simulink model "test_com_TireLoadEstimator"  (R2017a)
settings: Solver=FixedStepDiscrete  StartTime=450  StopTime=650  FixedStep=0.001  RelTol=1e-3
undefined symbols (not defined in the file or in its folder): GearRatio
settings Model: DataDictionary=controller_dict.sldd  SnapshotInterval=100  Creator=daniel  LastModifiedBy=rieth
settings DataIOCC: ExternalInput=VD_SteeringAngle_Value, VD_V2O_SpeedLongitudinal, VD_V2O_SpeedLateral, PT_Motor_MotorSpeed_FL, PT_Motor_MotorSpeed_FR, PT_Motor_MotorSpeed_RL, PT_Motor_MotorSpeed_RR, VD_Gyro_Front_Accel_X, VD_Gyro_Front_Accel_Y, VD_Gyro_Front_Accel_Z, VD_Gyro_Front_ARate_X, VD_Gyro_Front_ARate_Y, VD_Gyro_Front_ARate_Z, VD_Gyro_Front_Comp_X, VD_Gyro_Front_Comp_Y, VD_Gyro_Front_Comp_Z, VD_Gyro_Front_Temp, VD_Gyro_Rear_Accel_X, VD_Gyro_Rear_Accel_Y, VD_Gyro_Rear_Accel_Z, VD_Gyro_Rear_ARate_X, VD_Gyro_Rear_ARate_Y,VD_Gyro_Rear_ARate_Z, VD_Gyro_Rear_Comp_X, VD_Gyro_Rear_Comp_Y, VD_Gyro_Rear_Comp_Z, VD_Gyro_Rear_Temp,VD_Suspension_Hall_FL,VD_Suspension_Hall_FR,VD_Suspension_Hall_RL,VD_Suspension_Hall_RR  LimitDataPoints=on  LoadExternalInput=on  SaveFormat=Array  SaveOutput=off  SignalLogging=off  DSMLogging=off  SaveTime=off
settings OptimizationCC: DefaultParameterBehavior=Inlined  UseDivisionForNetSlopeComputation=on  StateBitsets=on  DataBitsets=on  LifeSpan=1
settings DebuggingCC: SolverPrmCheckMsg=warning  ParameterPrecisionLossMsg=none  AllowSymbolicDim=off  SFUnexpectedBacktrackingDiag=warning  SFNoUnconditionalDefaultTransitionDiag=warning  SFExecutionAtInitializationDiag=none
settings HardwareCC: ProdBitPerPointer=32  ProdBitPerSizeT=32  ProdBitPerPtrDiffT=32  ProdLargestAtomicInteger=Long  ProdLargestAtomicFloat=Double  ProdWordSize=32  ProdHWDeviceType=Texas Instruments->TMS570 Cortex-R4
settings ModelReferenceCC: PropagateSignalLabelsOutOfModel=off
settings SFSimCC: SimBuildMode=sf_nonincremental_build  MATLABDynamicMemAlloc=off
settings RTWCC: SystemTargetFile=ert.tlc  GenCodeOnly=on  TemplateMakefile=ert_default_tmf  Description=Embedded Coder  GenerateReport=on  BuildConfiguration=Faster Runs  IncludeHyperlinkInReport=on  LaunchReport=on  GenerateTraceReport=on
settings CodeAppCC: IgnoreCustomStorageClasses=off  SFDataObjDesc=on
settings ERTTargetCC: MultiwordLength=2048  GenerateSampleERTMain=on  InlinedParameterPlacement=NonHierarchical  ERTCustomFileTemplate=example_file_process.tlc  ConvertIfToSwitch=off  SuppressUnreachableDefaultCases=off
settings ConfigComp: CovMetricSettings=dw  CovHtmlReporting=on  CovSaveCumulativeToWorkspaceVar=on  CovSaveSingleToWorkspaceVar=on  CovExternalEMLEnable=off  CovSFcnEnable=off
settings ConfigurationSet: Description=SimMechanics 2G

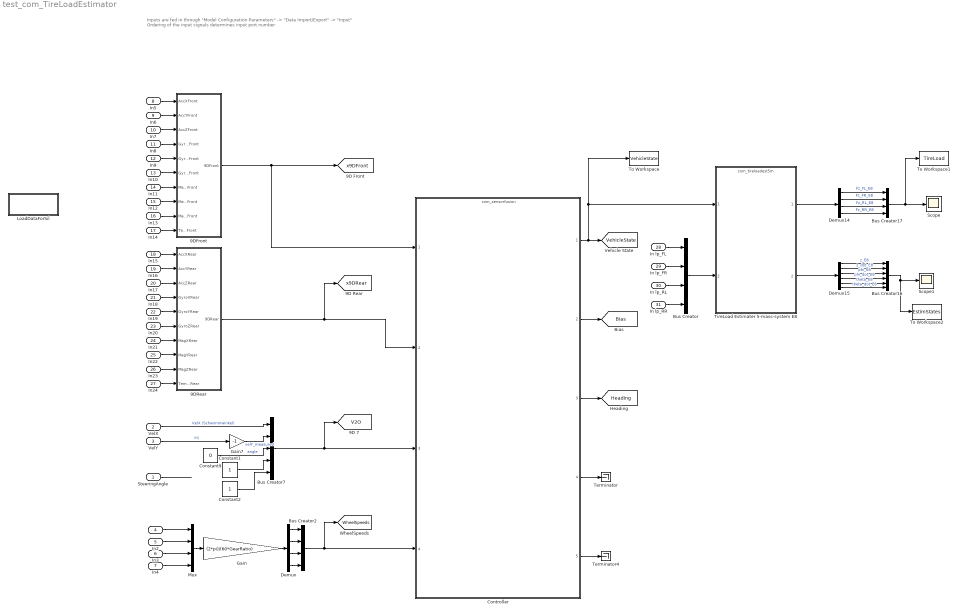
== system test_com_TireLoadEstimator ==
  note: Inputs are fed in through "Model Configuration Parameters" -> "Data Import/Export" -> "Input"
      | Ordering of the input signals determines input port number
  SteeringAngle : Inport  OutDataTypeStr=single  Interpolate=off
  VelX : Inport  Port=2  OutDataTypeStr=single
  VelY : Inport  Port=3  OutDataTypeStr=single
  " " : Inport  Port=4  OutDataTypeStr=single
  In2 : Inport  Port=5  OutDataTypeStr=single
  In3 : Inport  Port=6  OutDataTypeStr=single
  In4 : Inport  Port=7  OutDataTypeStr=single
  In5 : Inport  Port=8
  In6 : Inport  Port=9
  In7 : Inport  Port=10
  In8 : Inport  Port=11
  In9 : Inport  Port=12
  In10 : Inport  Port=13
  In11 : Inport  Port=14
  In12 : Inport  Port=15
  In13 : Inport  Port=16
  In14 : Inport  Port=17
  In15 : Inport  Port=18
  In16 : Inport  Port=19
  In17 : Inport  Port=20
  In18 : Inport  Port=21
  In19 : Inport  Port=22
  In20 : Inport  Port=23
  In21 : Inport  Port=24
  In22 : Inport  Port=25
  In23 : Inport  Port=26
  In24 : Inport  Port=27
  In lp_FL : Inport  Port=28  OutDataTypeStr=single
  In lp_FR : Inport  Port=29  OutDataTypeStr=single
  In lp_RL : Inport  Port=30  OutDataTypeStr=single
  In lp_RR : Inport  Port=31  OutDataTypeStr=single
  9DFront : Subsystem
  9DRear : Subsystem
  Bus Creator : BusCreator  Inputs=4
  Bus Creator16 : BusCreator  Inputs=6
  Bus Creator17 : BusCreator  Inputs=4
  Bus Creator2 : BusCreator  Inputs=4  OutDataTypeStr=Bus: control_WheelSpeed
      settings: InheritFromInputs=off
  Bus Creator7 : BusCreator  Inputs=5  OutDataTypeStr=Bus: control_velocity
      settings: InheritFromInputs=off
  Constant1 : Constant  OutDataTypeStr=boolean
  Constant2 : Constant  OutDataTypeStr=boolean
  Constant9 : Constant  Value=0  OutDataTypeStr=Inherit: Inherit via back propagation
  Controller : ModelReference  ModelNameDialog=com_sensorfusion.slx  SimulationMode=Normal  ModelReferenceVersion=1.1509
  Demux : Demux
  Demux14 : Demux
  Demux15 : Demux  Outputs=6
  Gain : Gain  Gain=(2*pi)/(60*GearRatio)
  Gain7 : Gain  Gain=-1
  LoadDataForSil : Subsystem
      settings: OpenFcn=LoadDataForSil
  Mux : Mux
  Scope : Scope
  Scope1 : Scope
  Terminator : Terminator
  Terminator4 : Terminator
  TireLoad Estimater 5-mass-system E8 : ModelReference  ModelNameDialog=com_tireloadest5m.slx  SimulationMode=Normal  ModelReferenceVersion=1.119
  To Workspace : ToWorkspace  VariableName=VehicleState  SaveFormat=Structure With Time  SampleTime=-1
  To Workspace1 : ToWorkspace  VariableName=TireLoad  SaveFormat=Structure With Time  SampleTime=-1
  To Workspace2 : ToWorkspace  VariableName=EstimStates  SaveFormat=Structure With Time  SampleTime=-1
  tag scope: Bias=global, Heading=global, V2O=global, VehicleState=global, WheelSpeeds=global, x9DFront=global, x9DRear=global
  wires:
  Bus Creator7/1 -> [V2O], Controller/3
  9DRear/1(9DRear) -> Controller/2, [x9DRear]
  VelY/1 -> Gain7/1  "vq"
  Constant9/1 -> Bus Creator7/3  "angle"
  Demux/1 -> Bus Creator2/1
  Demux/2 -> Bus Creator2/2
  Demux/3 -> Bus Creator2/3
  Gain/1 -> Demux/1
  Mux/1 -> Gain/1
  " "/1 -> Mux/1
  In2/1 -> Mux/2
  In3/1 -> Mux/3
  In4/1 -> Mux/4
  VelX/1 -> Bus Creator7/1  "VelX (Schwimmwinkel)"
  SteeringAngle/1 -> ?
  Gain7/1 -> Bus Creator7/2  "velY_measured"
  Demux/4 -> Bus Creator2/4
  In5/1 -> 9DFront/1(AccXFront)
  In6/1 -> 9DFront/2(AccYFront)
  In7/1 -> 9DFront/3(AccZFront)
  In8/1 -> 9DFront/4(GyroXFront)
  In9/1 -> 9DFront/5(GyroYFront)
  In10/1 -> 9DFront/6(GyroZFront)
  In11/1 -> 9DFront/7(MagXFront)
  In12/1 -> 9DFront/8(MagYFront)
  In13/1 -> 9DFront/9(MagZFront)
  In14/1 -> 9DFront/10(Temp9DFront)
  In16/1 -> 9DRear/2(AccYRear)
  In18/1 -> 9DRear/4(GyroXRear)
  In21/1 -> 9DRear/7(MagXRear)
  In23/1 -> 9DRear/9(MagZRear)
  In19/1 -> 9DRear/5(GyroYRear)
  In24/1 -> 9DRear/10(Temp9DRear)
  In20/1 -> 9DRear/6(GyroZRear)
  In15/1 -> 9DRear/1(AccXRear)
  In22/1 -> 9DRear/8(MagYRear)
  In17/1 -> 9DRear/3(AccZRear)
  9DFront/1(9DFront) -> [x9DFront], Controller/1
  Controller/2 -> [Bias]
  Controller/3 -> [Heading]
  Controller/4 -> Terminator/1
  Bus Creator2/1 -> Controller/4, [WheelSpeeds]
  In lp_FL/1 -> Bus Creator/1
  In lp_FR/1 -> Bus Creator/2
  In lp_RL/1 -> Bus Creator/3
  In lp_RR/1 -> Bus Creator/4
  Bus Creator/1 -> TireLoad Estimater 5-mass-system E8/2
  Constant1/1 -> Bus Creator7/4
  Demux15/1 -> Bus Creator16/1  "z_E8"
  Demux15/6 -> Bus Creator16/6  "theta_dot_E8"
  Demux15/5 -> Bus Creator16/5  "theta_E8"
  Demux15/4 -> Bus Creator16/4  "phi_dot_E8"
  Demux15/3 -> Bus Creator16/3  "phi_E8"
  Demux15/2 -> Bus Creator16/2  "z_dot_E8"
  Demux14/1 -> Bus Creator17/1  "Fz_FL_E8"
  Demux14/2 -> Bus Creator17/2  "Fz_FR_E8"
  Demux14/3 -> Bus Creator17/3  "Fz_RL_E8"
  Demux14/4 -> Bus Creator17/4  "Fz_RR_E8"
  Controller/1 -> [VehicleState], To Workspace/1, TireLoad Estimater 5-mass-system E8/1
  TireLoad Estimater 5-mass-system E8/2 -> Demux15/1
  TireLoad Estimater 5-mass-system E8/1 -> Demux14/1
  Controller/5 -> Terminator4/1
  Constant2/1 -> Bus Creator7/5
  Bus Creator17/1 -> To Workspace1/1, Scope/1
  Bus Creator16/1 -> Scope1/1, To Workspace2/1

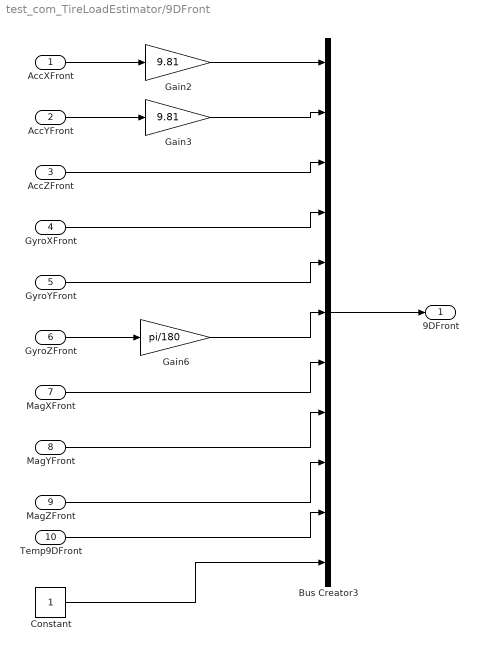
== system test_com_TireLoadEstimator/9DFront ==
  AccXFront : Inport
  AccYFront : Inport  Port=2
  AccZFront : Inport  Port=3
  GyroXFront : Inport  Port=4
  GyroYFront : Inport  Port=5
  GyroZFront : Inport  Port=6
  MagXFront : Inport  Port=7
  MagYFront : Inport  Port=8
  MagZFront : Inport  Port=9
  Temp9DFront : Inport  Port=10
  Bus Creator3 : BusCreator  Inputs=11  OutDataTypeStr=Bus: control_9D_Full_float
      settings: InheritFromInputs=off
  Constant : Constant  OutDataTypeStr=boolean
  Gain2 : Gain  Gain=9.81
  Gain3 : Gain  Gain=9.81
  Gain6 : Gain  Gain=pi/180
  9DFront : Outport
  wires:
  AccXFront/1 -> Gain2/1
  Temp9DFront/1 -> Bus Creator3/10
  GyroZFront/1 -> Gain6/1
  AccZFront/1 -> Bus Creator3/3
  AccYFront/1 -> Gain3/1
  GyroYFront/1 -> Bus Creator3/5
  MagZFront/1 -> Bus Creator3/9
  Gain2/1 -> Bus Creator3/1
  Bus Creator3/1 -> 9DFront/1
  MagYFront/1 -> Bus Creator3/8
  MagXFront/1 -> Bus Creator3/7
  Gain6/1 -> Bus Creator3/6
  GyroXFront/1 -> Bus Creator3/4
  Gain3/1 -> Bus Creator3/2
  Constant/1 -> Bus Creator3/11

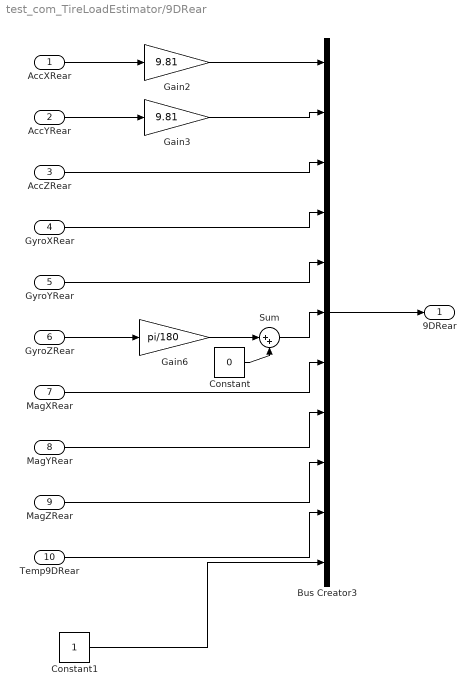
== system test_com_TireLoadEstimator/9DRear ==
  AccXRear : Inport
  AccYRear : Inport  Port=2
  AccZRear : Inport  Port=3
  GyroXRear : Inport  Port=4
  GyroYRear : Inport  Port=5
  GyroZRear : Inport  Port=6
  MagXRear : Inport  Port=7
  MagYRear : Inport  Port=8
  MagZRear : Inport  Port=9
  Temp9DRear : Inport  Port=10
  Bus Creator3 : BusCreator  Inputs=11  OutDataTypeStr=Bus: control_9D_Full_float
      settings: InheritFromInputs=off
  Constant : Constant  Value=0  OutDataTypeStr=single
  Constant1 : Constant  OutDataTypeStr=boolean
  Gain2 : Gain  Gain=9.81
  Gain3 : Gain  Gain=9.81
  Gain6 : Gain  Gain=pi/180
  Sum : Sum  Inputs=|++
  9DRear : Outport
  wires:
  GyroXRear/1 -> Bus Creator3/4
  Gain6/1 -> Sum/1
  MagXRear/1 -> Bus Creator3/7
  MagYRear/1 -> Bus Creator3/8
  Bus Creator3/1 -> 9DRear/1
  Gain3/1 -> Bus Creator3/2
  Gain2/1 -> Bus Creator3/1
  MagZRear/1 -> Bus Creator3/9
  GyroYRear/1 -> Bus Creator3/5
  AccYRear/1 -> Gain3/1
  AccZRear/1 -> Bus Creator3/3
  GyroZRear/1 -> Gain6/1
  Temp9DRear/1 -> Bus Creator3/10
  AccXRear/1 -> Gain2/1
  Sum/1 -> Bus Creator3/6
  Constant/1 -> Sum/2
  Constant1/1 -> Bus Creator3/11

== system test_com_TireLoadEstimator/LoadDataForSil ==
